simulink model "project_model_part2_chisquare"  (R2023a)
settings: Solver=VariableStepAuto  StartTime=0.0  StopTime=350  RelTol=1e-3
undefined symbols (not defined in the file): Discrete, Time
libraries: ctrlSharedLib x1
settings Model: Creator=Admin  LastModifiedBy=徐浩洋
settings SolverCC: AlgebraicLoopSolver=TrustRegion
settings DataIOCC: ReturnWorkspaceOutputs=off
settings DebuggingCC: UnconnectedInputMsg=warning  UnconnectedOutputMsg=warning  UnconnectedLineMsg=warning  ArithmeticOperatorsInVariantConditions=warning
settings ModelReferenceCC: EnableRefExpFcnMdlSchedulingChecks=on
settings SFSimCC: SimUseLocalCustomCode=off  CustomCodeUndefinedFunction=UseInterfaceOnly
settings RTWCC: RTWUseLocalCustomCode=off

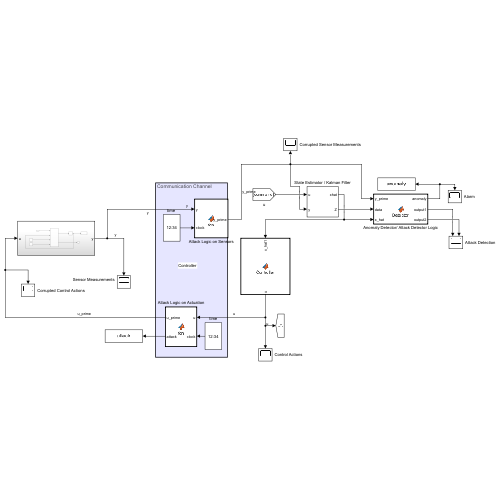
[thumbnail: Simulink's stored preview of the top-level diagram]
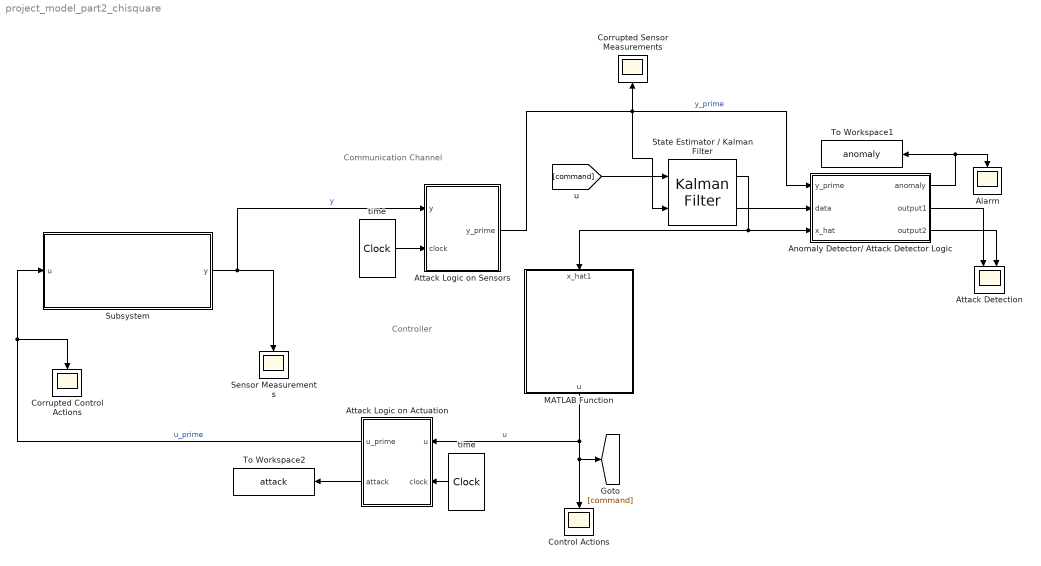
== system project_model_part2_chisquare ==
  note: Controller
  note: Communication Channel
  Alarm : Scope
  Anomaly Detector/ Attack Detector Logic : MATLAB Function  TreatAsAtomicUnit=on
  Attack Detection : Scope  NumInputPorts=2
  Attack Logic on Actuation : MATLAB Function  TreatAsAtomicUnit=on
  Attack Logic on Sensors : MATLAB Function  TreatAsAtomicUnit=on
  Control Actions : Scope
  Corrupted Control Actions : Scope
  Corrupted Sensor Measurements : Scope
  MATLAB Function : MATLAB Function  TreatAsAtomicUnit=on
  "Sensor Measurements " : Scope
  State Estimator / Kalman Filter : ctrlSharedLib/Kalman Filter  TimeDomain=Discrete-Time  UseCurrentEstimator=on  ModelSource=Individual A, B, C, D matrices  ModelSourceVariable=sys  A="[1.0000    0.0001   -0.0010;0.5747    1.0000   -0.0003;0.0162    0.0000    1.0000]"  B="[0.1   -0.2; -0.0536    0.0332;0.1955   -0.5294];"  C=[1 0 0;0 1 0]  D=[0 0;0 0]  NumberOfStates=2  NumberOfInputs=2  NumberOfOutputs=2  InitialEstimateSource=Dialog  X0=[0;0;0]  P0=10  UseK=off  UseGH=off  NumberOfProcessNoiseInputs=2  G=1  TimeInvariantG=on  H=0  TimeInvariantH=on  Q=0.00001*eye(3)  TimeInvariantQ=on  R=0.00008*eye(2)  TimeInvariantR=on  N=0  TimeInvariantN=on  AddInputPort=on  AddEnablePort=off  OutputEstimatedY=off  OutputP=on  Ts=-1
  Subsystem : Subsystem
  To Workspace1 : ToWorkspace  VariableName=anomaly  SaveFormat=Timeseries  SampleTime=0.1
      settings: Save2DSignal=2-D array (concatenate along first dimension)
  To Workspace2 : ToWorkspace  VariableName=attack  SaveFormat=Timeseries  SampleTime=0.1
      settings: Save2DSignal=2-D array (concatenate along first dimension)
  time : DigitalClock  SampleTime=0.1
  "time " : DigitalClock  SampleTime=0.1
  wires:
  "time "/1 -> Attack Logic on Sensors/2(clock)
  Attack Logic on Sensors/1(y_prime) -> State Estimator / Kalman Filter/2, Corrupted Sensor Measurements/1, Anomaly Detector/ Attack Detector Logic/1(y_prime)  "y_prime"
  MATLAB Function/1(u) -> Control Actions/1, [command], Attack Logic on Actuation/1(u)  "u"
  time/1 -> Attack Logic on Actuation/2(clock)
  Attack Logic on Actuation/1(u_prime) -> Subsystem/1(u), Corrupted Control Actions/1  "u_prime"
  [command] -> State Estimator / Kalman Filter/1
  Subsystem/1(y) -> Attack Logic on Sensors/1(y), "Sensor Measurements "/1  "y"
  State Estimator / Kalman Filter/1 -> MATLAB Function/1(x_hat1), Anomaly Detector/ Attack Detector Logic/3(x_hat)
  State Estimator / Kalman Filter/2 -> Anomaly Detector/ Attack Detector Logic/2(data)
  Anomaly Detector/ Attack Detector Logic/1(anomaly) -> Alarm/1, To Workspace1/1
  Anomaly Detector/ Attack Detector Logic/2(output1) -> Attack Detection/1
  Anomaly Detector/ Attack Detector Logic/3(output2) -> Attack Detection/2
  Attack Logic on Actuation/2(attack) -> To Workspace2/1

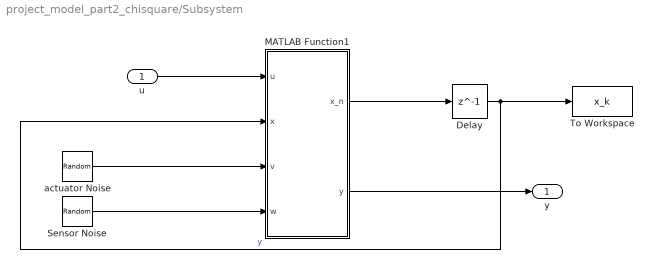
== system project_model_part2_chisquare/Subsystem ==
  u : Inport
  Delay : Delay  DelayLength=1  InitialCondition=[0 0.1 0.2]
  MATLAB Function1 : MATLAB Function  TreatAsAtomicUnit=on
  Sensor Noise : RandomNumber  Mean=[0 0]  Variance=[0.00008 0.00008]  Seed=[randi(100) randi(100)]
  To Workspace : ToWorkspace  VariableName=x_k  SaveFormat=Timeseries  SampleTime=-1
  actuator Noise : RandomNumber  Mean=[0 0 0]  Variance=[0.00001 0.00001 0.00001]  Seed=[randi(100) randi(100) randi(100)]
  y : Outport  VectorParamsAs1DForOutWhenUnconnected=off
  wires:
  u/1 -> MATLAB Function1/1(u)
  MATLAB Function1/1(x_n) -> Delay/1
  MATLAB Function1/2(y) -> y/1
  Sensor Noise/1 -> MATLAB Function1/4(w)
  actuator Noise/1 -> MATLAB Function1/3(v)
  Delay/1 -> To Workspace/1, MATLAB Function1/2(x)  "y"

== matlab function project_model_part2_chisquare/Attack Logic on Sensors ==
  data: y input; y_prime output; clock input
function y_prime = fcn(y,clock)
% this function should contain the attacker action on the sensor
% measurements
y_prime = y;
end

== matlab function project_model_part2_chisquare/MATLAB Function ==
  data: x_hat1 input; u output
function u  = Controller(x_hat1)
%two tanks model 
    

%controller gain
K =[17.1291   -1.1789   -6.5335; -0.1248   -2.9385   -2.5082];
u=-K*(x_hat1);

== matlab function project_model_part2_chisquare/Attack Logic on Actuation ==
  data: u input; u_prime output; clock input; attack output
function [u_prime,attack] = fcn(u,clock)
% this function should contain the attacker action on the control inputs

%False data injection on Actuation Channel
if clock >= 0 && clock < 40
    u_a = transpose([0 ,0]);
    attack = 0;
elseif clock >= 40 && clock < 50
    u_a = transpose([-0.18 ,-0.18]);
    attack = 1;
elseif clock >= 50 && clock < 300
    u_a = transpose([0 ,0]);
    attack = 0;
elseif clock >= 300 && clock < 310
    u_a = transpose([-0.21 ,-0.21]);
    attack = 1;
else
    u_a = transpose([0 ,0]);
    attack = 0;
end
u_prime = u + u_a;

end

== matlab function project_model_part2_chisquare/Anomaly Detector// Attack Detector Logic ==
  data: y_prime input; data input; x_hat input; anomaly output; output1 output; output2 output
function [anomaly ,output1 ,output2] = Detector(y_prime , data, x_hat)
% this function should contain the detection strategy

% for the chi square detector "z" should be the name of detection signal and
% "tau" the name of threshold

% Chi-square detection algoritm
C = [1 0 0; 0 1 0];
R = 0.00008*eye(2);
P = data;
sigma = (C * P * (transpose(C))) + R;
r = y_prime - (C * x_hat);
% Detection signal
z = transpose(r) * (inv(sigma) * r);
alpha = 0.09;
v = size(r);
% Threshold
tau = chi2inv(1-alpha , v);
if z <= tau
    alarm = 'NO';
    anomaly = 0;
else
    alarm = 'YES';
    anomaly = 1;
end
output1 = z;
output2 = tau;
end

== matlab function project_model_part2_chisquare/Subsystem/MATLAB Function1 ==
  data: x_n output; u input; y output; x input; v input; w input
function [x_n, y] = fcn(u, x, v, w)

A=[1.0000    0.0001   -0.0010;0.5747    1.0000   -0.0003;0.0162    0.0000    1.0000];
B = [0.1   -0.2; -0.0536    0.0332;0.1955   -0.5294];

C=[1 0 0;0 1 0];
D=[0 0;0 0];


x_n = A*x + B*u + v;
y = C*x + D*u + w;
